simulink model "alpha_hat"  (R2015b)
settings: Solver=VariableStepAuto  StartTime=0.0  StopTime=10.0  RelTol=1e-3
settings Model: Creator=yuji  LastModifiedBy=yuji

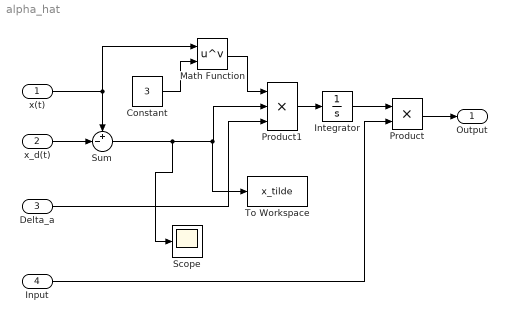
== system alpha_hat ==
  x(t) : Inport
  x_d(t) : Inport  Port=2
  Delta_a : Inport  Port=3
  Input : Inport  Port=4
  Constant : Constant  Value=3
  Integrator : Integrator
  Math Function : Math  Operator=pow  SaturateOnIntegerOverflow=on
  Product : Product
  Product1 : Product  Inputs=3
  Scope : Scope
  Sum : Sum  Inputs=+-|
  To Workspace : ToWorkspace  VariableName=x_tilde  SaveFormat=Timeseries  SampleTime=-1
  Output : Outport
  wires:
  Product/1 -> Output/1
  Input/1 -> Product/2
  Integrator/1 -> Product/1
  Product1/1 -> Integrator/1
  Delta_a/1 -> Product1/3
  x_d(t)/1 -> Sum/2
  Sum/1 -> To Workspace/1, Product1/2, Scope/1
  x(t)/1 -> Sum/1, Math Function/1
  Constant/1 -> Math Function/2
  Math Function/1 -> Product1/1
